simulink model "ESTS_VHSO_test"  (R2023b)
settings: Solver=VariableStepAuto  StartTime=0.0  StopTime=10.0  RelTol=1e-3
libraries: ESTS_VHSO x1, simulink x1
settings Model: Creator=blatak  LastModifiedBy=blatak

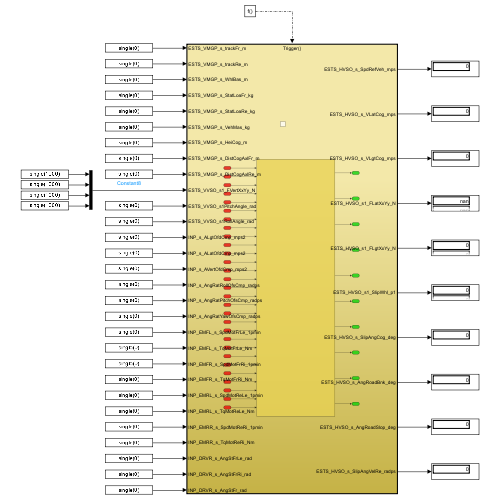
[thumbnail: Simulink's stored preview of the top-level diagram]
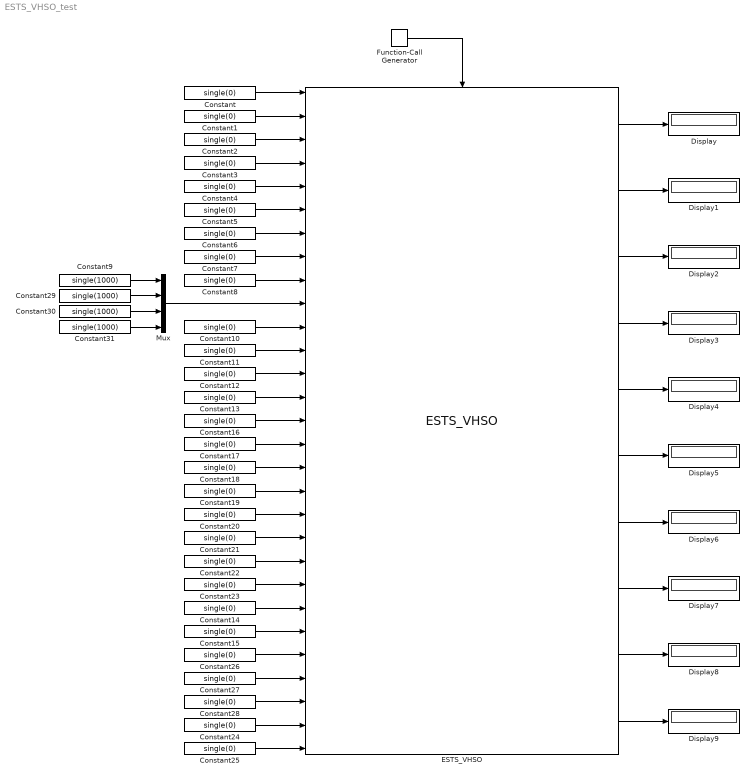
== system ESTS_VHSO_test ==
  Constant{,1..8,10..28} (28 alike) : Constant  Value=single(0)
  Constant{9,29..31} (4 alike) : Constant  Value=single(1000)
  Display{,1..9} (10 alike) : Display
  ESTS_VHSO : ESTS_VHSO/ESTS_VHSO  SystemSampleTime=-1  VariantActivationTime=update diagram  AllowFlexibleInterface=on  Latency=0  AutoFrameSizeCalculation=off
  Function-Call Generator : simulink/Ports & Subsystems/Function-Call Generator  sample_time=0.01  numberOfIterations=1  DisallowWideOutput=off
  Mux : Mux
  wires:
  Function-Call Generator/1 -> ESTS_VHSO/Trigger
  Constant/1 -> ESTS_VHSO/1
  Constant1/1 -> ESTS_VHSO/2
  Constant2/1 -> ESTS_VHSO/3
  Constant3/1 -> ESTS_VHSO/4
  Constant4/1 -> ESTS_VHSO/5
  Constant5/1 -> ESTS_VHSO/6
  Constant6/1 -> ESTS_VHSO/7
  Constant7/1 -> ESTS_VHSO/8
  Constant8/1 -> ESTS_VHSO/9
  Mux/1 -> ESTS_VHSO/10
  Constant10/1 -> ESTS_VHSO/11
  Constant11/1 -> ESTS_VHSO/12
  Constant12/1 -> ESTS_VHSO/13
  Constant13/1 -> ESTS_VHSO/14
  Constant16/1 -> ESTS_VHSO/15
  Constant17/1 -> ESTS_VHSO/16
  Constant18/1 -> ESTS_VHSO/17
  Constant19/1 -> ESTS_VHSO/18
  Constant20/1 -> ESTS_VHSO/19
  Constant21/1 -> ESTS_VHSO/20
  Constant22/1 -> ESTS_VHSO/21
  Constant23/1 -> ESTS_VHSO/22
  Constant14/1 -> ESTS_VHSO/23
  Constant15/1 -> ESTS_VHSO/24
  Constant26/1 -> ESTS_VHSO/25
  Constant27/1 -> ESTS_VHSO/26
  Constant28/1 -> ESTS_VHSO/27
  Constant24/1 -> ESTS_VHSO/28
  Constant25/1 -> ESTS_VHSO/29
  ESTS_VHSO/1 -> Display/1
  ESTS_VHSO/2 -> Display1/1
  ESTS_VHSO/3 -> Display2/1
  ESTS_VHSO/4 -> Display3/1
  ESTS_VHSO/5 -> Display4/1
  ESTS_VHSO/6 -> Display5/1
  ESTS_VHSO/7 -> Display6/1
  ESTS_VHSO/8 -> Display7/1
  ESTS_VHSO/9 -> Display8/1
  ESTS_VHSO/10 -> Display9/1
  Constant9/1 -> Mux/1
  Constant29/1 -> Mux/2
  Constant30/1 -> Mux/3
  Constant31/1 -> Mux/4
